simulink model "Op_Space_Compliance_Control"  (R2020b)
settings: Solver=VariableStepAuto  StartTime=0.0  StopTime=10  RelTol=1e-3
values from neighbouring files (symbols this model uses):
  G = myRobot.G_Lagrangian    [hw11_main.m]
  J = myRobot.J    [hw11_main.m]
  K = diag([1,10,1,0,0,0])    [hw11_main.m]
  Kd = diag([24,15,15,0,0,0])    [hw11_main.m]
  Kp = diag([28,22,20,0,0,0])    [hw11_main.m]
  T_d = [R_d, x_d(1:3); [0 0 0 1]]    [hw11_main.m]
  x_d = [0.3 ; 0.5; 0.8; -pi/2; -pi/2; -pi/2]    [hw11_main.m]
  x_r = [0.8;0.52; 0.3; -pi/2; -pi/2; -pi/2]    [hw11_main.m]
settings Model: Creator=nicol  LastModifiedBy=nicol

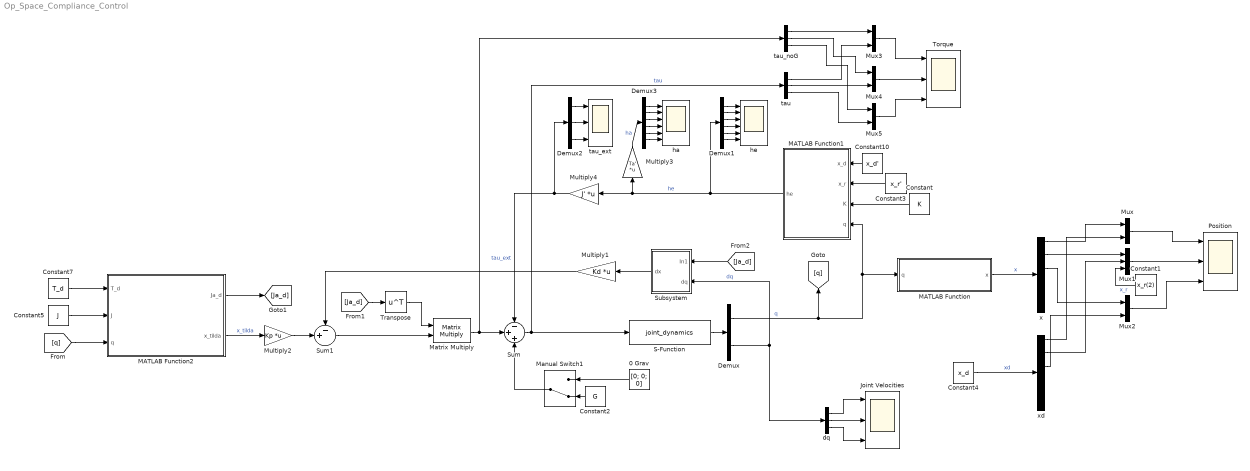
== system Op_Space_Compliance_Control ==
  0 Grav : Constant  Value=[0; 0; 0]  VectorParams1D=off
  Constant : Constant  Value=K
  Constant1 : Constant  Value=x_r(2)
  Constant10 : Constant  Value=x_d'
  Constant2 : Constant  Value=G  VectorParams1D=off
  Constant3 : Constant  Value=x_r'
  Constant4 : Constant  Value=x_d  VectorParams1D=off
  Constant5 : Constant  Value=J
  Constant7 : Constant  Value=T_d
  Demux : Demux  Outputs=2
  Demux1 : Demux  Outputs=6
  Demux2 : Demux  Outputs=3
  Demux3 : Demux  Outputs=6
  Joint Velocities : Scope  NumInputPorts=3
  MATLAB Function : MATLAB Function  TreatAsAtomicUnit=on
  MATLAB Function1 : MATLAB Function  TreatAsAtomicUnit=on
  MATLAB Function2 : MATLAB Function  TreatAsAtomicUnit=on
  Manual Switch1 : ManualSwitch  CurrentSetting=0
  Matrix Multiply : Product  Multiplication=Matrix(*)
  Multiply1 : Gain  Gain=Kd  Multiplication=Matrix(K*u)
  Multiply2 : Gain  Gain=Kp  Multiplication=Matrix(K*u)
  Multiply3 : Gain  Gain=Ta'  Multiplication=Matrix(K*u)
  Multiply4 : Gain  Gain=J'  Multiplication=Matrix(K*u)
  Mux{,2..5} (5 alike) : Mux  Inputs=2
  Mux1 : Mux  Inputs=3
  Position : Scope  NumInputPorts=3
  S-Function : S-Function  FunctionName=joint_dynamics  Parameters=myRobot  SFunctionDeploymentMode=off  EnableBusSupport=off
  Subsystem : Subsystem
  Sum : Sum  Inputs=-++
  Sum1 : Sum  Inputs=-+|
  Torque : Scope  NumInputPorts=3
  Transpose : Math  Operator=transpose  SaturateOnIntegerOverflow=on
  dq : Demux  Outputs=3
  ha : Scope  NumInputPorts=6
  he : Scope  NumInputPorts=6
  tau : Demux  Outputs=3
  tau_ext : Scope  NumInputPorts=3
  tau_noG : Demux  Outputs=3
  x : Demux  Outputs=6
  xd : Demux  Outputs=6
  wires:
  Constant2/1 -> Manual Switch1/2
  Manual Switch1/1 -> Sum/3
  0 Grav/1 -> Manual Switch1/1
  Multiply1/1 -> Sum1/1
  Multiply2/1 -> Sum1/2
  Constant4/1 -> xd/1  "xd"
  S-Function/1 -> Demux/1
  x/1 -> Mux/1
  x/3 -> Mux2/1
  Mux/1 -> Position/1
  Mux1/1 -> Position/2
  Mux2/1 -> Position/3
  dq/2 -> Joint Velocities/2
  dq/1 -> Joint Velocities/1
  dq/3 -> Joint Velocities/3
  Demux/2 -> Subsystem/2(dq), dq/1  "dq"
  Sum1/1 -> Matrix Multiply/2
  Demux/1 -> MATLAB Function/1(q), MATLAB Function1/4(q), [q]  "q"
  MATLAB Function/1(x) -> x/1  "x"
  tau/2 -> Mux4/2
  tau/3 -> Mux5/2
  Mux4/1 -> Torque/2
  Mux3/1 -> Torque/1
  Mux5/1 -> Torque/3
  tau_noG/1 -> Mux3/1
  tau_noG/2 -> Mux4/1
  tau/1 -> Mux3/2
  tau_noG/3 -> Mux5/1
  Constant/1 -> MATLAB Function1/3(K)
  MATLAB Function1/1(he) -> Multiply4/1, Multiply3/1, Demux1/1  "he"
  [q] -> MATLAB Function2/3(q)
  Constant5/1 -> MATLAB Function2/2(J)
  MATLAB Function2/1(Ja_d) -> [Ja_d]
  [Ja_d] -> Transpose/1
  Transpose/1 -> Matrix Multiply/1
  xd/1 -> Mux/2
  xd/2 -> Mux1/2
  xd/3 -> Mux2/2
  Constant7/1 -> MATLAB Function2/1(T_d)
  Constant3/1 -> MATLAB Function1/2(x_r)
  Demux1/1 -> he/1
  Demux1/2 -> he/2
  Demux1/3 -> he/3
  Demux1/4 -> he/4
  Demux1/5 -> he/5
  Demux1/6 -> he/6
  Sum/1 -> S-Function/1, tau/1  "tau"
  Multiply4/1 -> Sum/1, Demux2/1  "tau_ext"
  Demux2/3 -> tau_ext/3
  Demux2/2 -> tau_ext/2
  Demux2/1 -> tau_ext/1
  Demux3/1 -> ha/1
  Demux3/6 -> ha/6
  Demux3/2 -> ha/2
  Demux3/3 -> ha/3
  Demux3/4 -> ha/4
  Demux3/5 -> ha/5
  Multiply3/1 -> Demux3/1  "ha"
  Matrix Multiply/1 -> Sum/2, tau_noG/1
  MATLAB Function2/2(x_tilda) -> Multiply2/1  "x_tilda"
  [Ja_d] -> Subsystem/1(In1)
  Subsystem/1(dx) -> Multiply1/1
  x/2 -> Mux1/1
  Constant1/1 -> Mux1/3  "x_r"
  Constant10/1 -> MATLAB Function1/1(x_d)

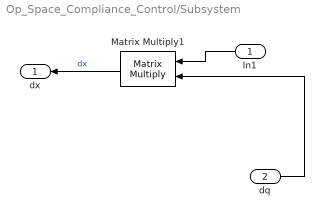
== system Op_Space_Compliance_Control/Subsystem ==
  In1 : Inport
  dq : Inport  Port=2
  Matrix Multiply1 : Product  Multiplication=Matrix(*)
  dx : Outport
  wires:
  In1/1 -> Matrix Multiply1/1
  Matrix Multiply1/1 -> dx/1  "dx"
  dq/1 -> Matrix Multiply1/2

== matlab function Op_Space_Compliance_Control/MATLAB Function1 ==
  data: x_d input; x_r input; K input; q input; he output
function he = Environment(x_d,x_r,K,q)

T_e=getTe(q);
x_e=zeros(6,1);
x_e(1:3,1)=T_e(1:3,4);
eul_e = rotm2eul(T_e(1:3,1:3),'ZYZ');
x_e(4:6,1)=eul_e;

if(x_e(2,1)-x_r(2,1)<0)
    he=[0;0;0;0;0;0];
else
    sup=zeros(6,1);
    dx_r_d=x_d-x_r;
    dx_e_d=x_d-x_e;
    sup(2,1)=dx_r_d(2,1)-dx_e_d(2,1);
    he=K*sup;
end

== matlab function Op_Space_Compliance_Control/MATLAB Function ==
  data: q input size=3; x output size=6
function x = directKinematics6Dof(q)
%last 3 components assigned constant since robot does not have rotational
%joints

x=[ q(1) + 1/5;
    q(3) + 1/5;
    q(2) + 1251/5000;
    -pi/2;
    -pi/2;
    -pi/2];
end

== matlab function Op_Space_Compliance_Control/MATLAB Function2 ==
  data: T_d input; J input; q input; Ja_d output; x_tilda output
function [Ja_d,x_tilda]   =getJa_dAndXTilda(T_d,J,q)
% desired rotational matrix
R_d=T_d(1:3,1:3);

% end effector rotational matrix
T_e=getTe(q);
R_e=T_e(1:3,1:3);

% homogenous transf for end effector pose expressed in desired frame
T_e_d=pinv(T_d)*T_e;
R_e_d=T_e_d(1:3,1:3);
phi_e_d=rotm2eul(R_e_d,'ZYZ');
x_tilda=-[T_e_d(1:3,4);phi_e_d'];

Ta=getTa(phi_e_d(1),phi_e_d(2),phi_e_d(3));

% version of the textbook and works
Ja_d=pinv(Ta)*[R_d' zeros(3);zeros(3) R_d']*J;

end
